simulink model "Block_receive_and_send_data_with_Slant_Distances_8"  (R2012b)
settings: Solver=ode45  StartTime=0.0  StopTime=inf  RelTol=1e-3
libraries: etargetslib x2, dspnetwork x2
settings Model: Creator=cheki_000  LastModifiedBy=cheki_000

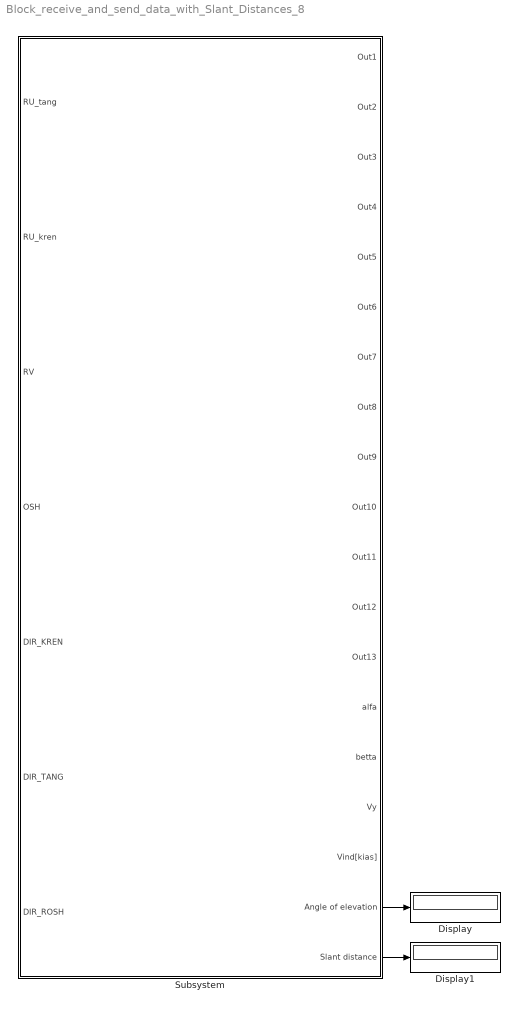
== system Block_receive_and_send_data_with_Slant_Distances_8 ==
  Display : Display
  Display1 : Display
  Subsystem : Subsystem
  wires:
  Subsystem/18(Angle of elevation) -> Display/1
  Subsystem/19(Slant distance) -> Display1/1

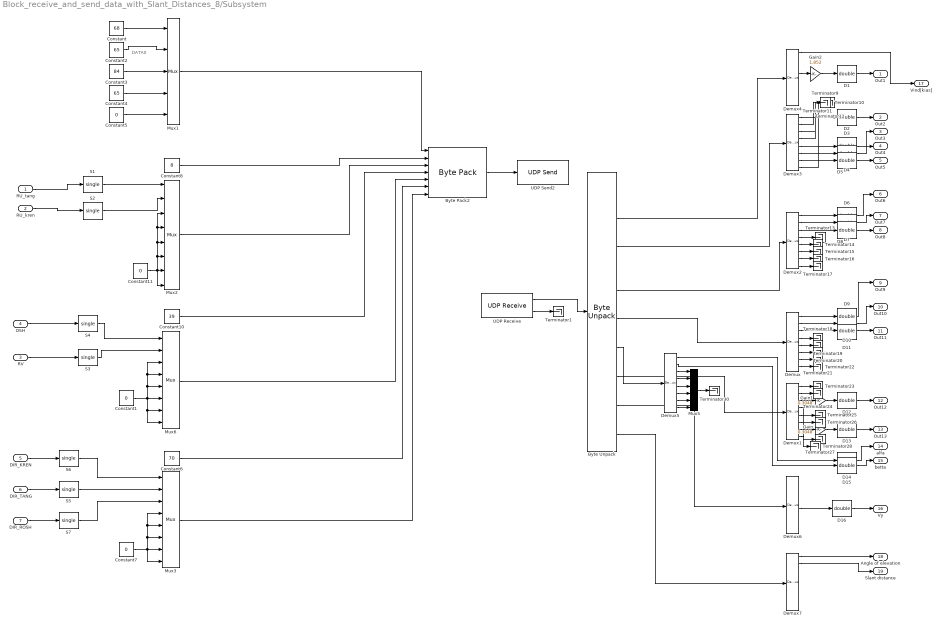
== system Block_receive_and_send_data_with_Slant_Distances_8/Subsystem ==
  note: DATA0
  RU_tang : Inport
  RU_kren : Inport  Port=2
  RV : Inport  Port=3
  OSH : Inport  Port=4
  DIR_KREN : Inport  Port=5
  DIR_TANG : Inport  Port=6
  DIR_ROSH : Inport  Port=7
  Byte Pack2 : etargetslib/Byte Pack  datatypes={'int8','int32','single','int32','single','int32','single'}  byteAlign=1
  Byte Unpack : etargetslib/Byte Unpack  dimensions={[5+3*36],[1],[8],[1],[8],[12*36],[1],[8],[1],[8],[1],[8],[1],[8],[1],[8],[1],[8]}  datatypes={'int8','int32','single','int32','single','int8','int32','single','int32','single','int32','single','int32','single','int32','single','int32','single'}  byteAlign=1
  Constant : Constant  Value=68  OutDataTypeStr=int8
  Constant1 : Constant  Value=0  OutDataTypeStr=single  LockScale=on
  Constant10 : Constant  Value=39  OutDataTypeStr=int32  LockScale=on
  Constant11 : Constant  Value=0  OutDataTypeStr=single  LockScale=on
  Constant2 : Constant  Value=65  OutDataTypeStr=int8  LockScale=on
  Constant3 : Constant  Value=84  OutDataTypeStr=int8
  Constant4 : Constant  Value=65  OutDataTypeStr=int8  LockScale=on
  Constant5 : Constant  Value=0  OutDataTypeStr=int8  LockScale=on
  Constant6 : Constant  Value=70  OutDataTypeStr=int32  LockScale=on
  Constant7 : Constant  Value=0  OutDataTypeStr=single  LockScale=on
  Constant8 : Constant  Value=8  OutDataTypeStr=int32  LockScale=on
  D{1..16} (16 alike) : DataTypeConversion  OutDataTypeStr=double
  Demux{,1..7} (8 alike) : Demux  Outputs=8
  Gain : Gain  Gain=0.3048
  Gain1 : Gain  Gain=0.3048
  Gain2 : Gain  Gain=1.852
  Mux1 : Mux  Inputs=5
  Mux2 : Mux  Inputs=8
  Mux3 : Mux  Inputs=8
  Mux5 : Mux  Inputs=6
  Mux6 : Mux  Inputs=8
  S{1..7} (7 alike) : DataTypeConversion  OutDataTypeStr=single
  Terminator{1,9..28,30} (22 alike) : Terminator
  UDP Receive : dspnetwork/UDP Receive  localURL='0.0.0.0'  localPort=4444  remoteURL='127.0.0.1'  remotePort=-1  recvBufferSize=8192  dims=720+5+36+36+36  signalDatatype=uint8  isVarSize=off  showBlockingTime=off  blockingTime=0  sampletime=inf
  UDP Send2 : dspnetwork/UDP Send  remoteURL='127.0.0.1'  remotePort=49000  localURL='0.0.0.0'  localPortSource=Automatically determine  localPort=4444  sampletime=-1  separateLengthPort=0
  Out1 : Outport
  Out2 : Outport  Port=2
  Out3 : Outport  Port=3
  Out4 : Outport  Port=4
  Out5 : Outport  Port=5
  Out6 : Outport  Port=6
  Out7 : Outport  Port=7
  Out8 : Outport  Port=8
  Out9 : Outport  Port=9
  Out10 : Outport  Port=10
  Out11 : Outport  Port=11
  Out12 : Outport  Port=12
  Out13 : Outport  Port=13
  alfa : Outport  Port=14
  betta : Outport  Port=15
  Vy : Outport  Port=16
  Vind[kias] : Outport  Port=17
  Angle of elevation : Outport  Port=18
  Slant distance : Outport  Port=19
  wires:
  Byte Pack2/1 -> UDP Send2/1
  Demux1/4 -> Gain/1
  Demux1/3 -> Gain1/1
  Byte Unpack/8 -> Demux2/1
  Byte Unpack/5 -> Demux3/1
  Demux4/4 -> Gain2/1
  Byte Unpack/3 -> Demux4/1
  Demux3/2 -> Terminator9/1
  Demux3/3 -> Terminator10/1
  Demux3/4 -> Terminator11/1
  Demux3/8 -> Terminator12/1
  Demux2/4 -> Terminator13/1
  Demux2/5 -> Terminator14/1
  Demux2/6 -> Terminator15/1
  Demux2/7 -> Terminator16/1
  Demux2/8 -> Terminator17/1
  Demux/4 -> Terminator18/1
  Demux/5 -> Terminator19/1
  Demux/6 -> Terminator20/1
  Demux/7 -> Terminator21/1
  Demux/8 -> Terminator22/1
  Demux1/1 -> Terminator23/1
  Demux1/2 -> Terminator24/1
  Demux1/5 -> Terminator25/1
  Demux1/6 -> Terminator26/1
  Demux1/7 -> Terminator27/1
  Demux1/8 -> Terminator28/1
  Gain2/1 -> D1/1
  Demux3/1 -> D2/1
  Demux3/5 -> D3/1
  Demux3/6 -> D4/1
  Demux3/7 -> D5/1
  Demux2/1 -> D6/1
  Demux2/2 -> D7/1
  Demux2/3 -> D8/1
  Demux/1 -> D9/1
  Demux/2 -> D10/1
  Demux/3 -> D11/1
  Gain1/1 -> D12/1
  Gain/1 -> D13/1
  D1/1 -> Out1/1
  D2/1 -> Out2/1
  D3/1 -> Out3/1
  D4/1 -> Out4/1
  D5/1 -> Out5/1
  D6/1 -> Out6/1
  D7/1 -> Out7/1
  D8/1 -> Out8/1
  D9/1 -> Out9/1
  D10/1 -> Out10/1
  D11/1 -> Out11/1
  D12/1 -> Out12/1
  D13/1 -> Out13/1
  Byte Unpack/12 -> Demux5/1
  Demux5/1 -> D14/1
  Demux5/2 -> D15/1
  Demux5/3 -> Mux5/1
  Demux5/4 -> Mux5/2
  Demux5/5 -> Mux5/3
  Demux5/6 -> Mux5/4
  Demux5/7 -> Mux5/5
  Demux5/8 -> Mux5/6
  Mux5/1 -> Terminator30/1
  D14/1 -> alfa/1
  D15/1 -> betta/1
  UDP Receive/1 -> Byte Unpack/1
  Byte Unpack/10 -> Demux/1
  Byte Unpack/14 -> Demux1/1
  UDP Receive/2 -> Terminator1/1
  Byte Unpack/16 -> Demux6/1
  Demux6/5 -> D16/1
  D16/1 -> Vy/1
  Constant/1 -> Mux1/1
  Constant2/1 -> Mux1/2
  Constant3/1 -> Mux1/3
  Constant4/1 -> Mux1/4
  Constant5/1 -> Mux1/5
  Mux1/1 -> Byte Pack2/1
  Constant8/1 -> Byte Pack2/2
  Mux2/1 -> Byte Pack2/3
  OSH/1 -> S4/1
  Constant11/1 -> Mux2/7, Mux2/3, Mux2/4, Mux2/5, Mux2/6, Mux2/8
  RU_tang/1 -> S1/1
  RU_kren/1 -> S2/1
  RV/1 -> S3/1
  S1/1 -> Mux2/1
  S2/1 -> Mux2/2
  S4/1 -> Mux6/1
  Constant10/1 -> Byte Pack2/4
  Constant1/1 -> Mux6/8, Mux6/7, Mux6/3, Mux6/4, Mux6/5, Mux6/6
  Mux6/1 -> Byte Pack2/5
  S3/1 -> Mux6/2
  Constant6/1 -> Byte Pack2/6
  DIR_KREN/1 -> S6/1
  DIR_TANG/1 -> S5/1
  DIR_ROSH/1 -> S7/1
  Mux3/1 -> Byte Pack2/7
  S6/1 -> Mux3/1
  S5/1 -> Mux3/2
  S7/1 -> Mux3/3
  Constant7/1 -> Mux3/7, Mux3/6, Mux3/5, Mux3/4, Mux3/8
  Demux4/1 -> Vind[kias]/1
  Demux7/1 -> Angle of elevation/1
  Demux7/2 -> Slant distance/1
  Byte Unpack/18 -> Demux7/1
